simulink model "MSZSZ_Inga"  (R2025a)
settings: Solver=VariableStepAuto  StartTime=0.0  StopTime=50  MaxStep=10e-3  RelTol=1e-3
libraries: simulink_extras x1
settings Model: Creator=Szalay  LastModifiedBy=Szalay

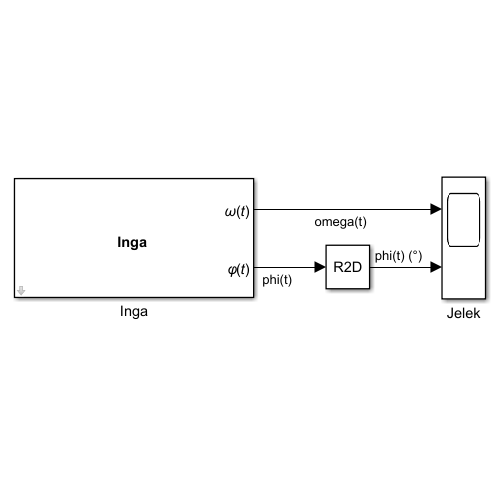
[thumbnail: Simulink's stored preview of the top-level diagram]
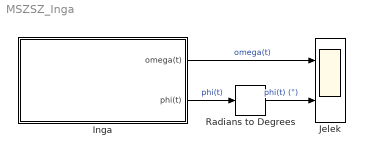
== system MSZSZ_Inga ==
  Inga : Subsystem  mask{m=1, L=1, g=9.81, B=0.2, omega_0=0, phi_0=deg2rad(45)}
      mask prompts: m "Tömeg"; L "Hossz"; g "Nehézségi térerő"; B "Forgási súrlódási együttható"; omega_0 "Kezdeti szögsebesség"; phi_0 "Kezdeti szöghelyzet"
      mask init:
      | J = m*L^2;
      mask DialogControl ParameterGroupVar Prompt: Modellparaméterek
      mask DialogControl Container3 Prompt: Kezdeti értékek
      mask Display:
      | % Kimenetek
      | port_label('output', 1, '{\it\omega}({\itt})', "Interpreter", "tex");
      | port_label('output', 2, '{\it\phi}({\itt})', "Interpreter", "tex");
      | 
      | text( ...
      |     0.5, 0.5, '{\bfInga}', ...
      |     'HorizontalAlignment', 'center', ...
      |     'Interpreter', 'tex' ...
      |     );
  Jelek : Scope  NumInputPorts=2
      settings: ActiveDisplayYMinimum=-2.8222054169075976  ActiveDisplayYMaximum=2.6012131657726636
  Radians to Degrees : simulink_extras/Transformations/Radians to Degrees
  wires:
  Inga/1(omega(t)) -> Jelek/1  "omega(t)"
  Radians to Degrees/1 -> Jelek/2  "phi(t) (°)"
  Inga/2(phi(t)) -> Radians to Degrees/1  "phi(t)"

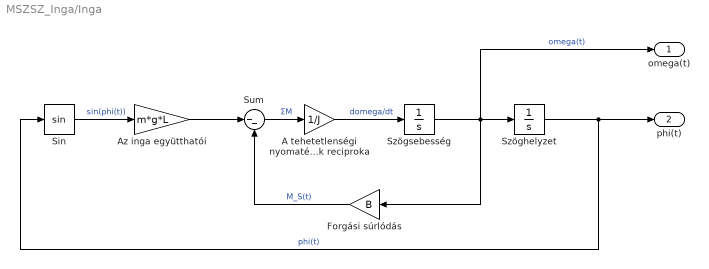
== system MSZSZ_Inga/Inga ==
  A tehetetlenségi nyomaték reciproka : Gain  Gain=1/J
  Az inga együtthatói : Gain  Gain=m*g*L
  Forgási súrlódás : Gain  Gain=B
  Sin : Trigonometry
  Sum : Sum  Inputs=|--
  Szöghelyzet : Integrator  InitialCondition=phi_0
  Szögsebesség : Integrator  InitialCondition=omega_0
  omega(t) : Outport
  phi(t) : Outport  Port=2
  wires:
  Sum/1 -> A tehetetlenségi nyomaték reciproka/1  "ΣM"
  A tehetetlenségi nyomaték reciproka/1 -> Szögsebesség/1  "domega/dt"
  Sin/1 -> Az inga együtthatói/1  "sin(phi(t))"
  Szögsebesség/1 -> omega(t)/1, Forgási súrlódás/1, Szöghelyzet/1  "omega(t)"
  Az inga együtthatói/1 -> Sum/1
  Szöghelyzet/1 -> phi(t)/1, Sin/1  "phi(t)"
  Forgási súrlódás/1 -> Sum/2  "M_S(t)"
